simulink model "TSR_Scenario_005_cs"  (R2014b)
settings: Solver=ode5  SolverMode=SingleTasking  StartTime=0.0  StopTime=inf  FixedStep=1/100  RelTol=1e-3
PreLoadFcn:
  | mbxruntime.callbacks.PreLoadFcn(bdroot);
  | check_NUTS_defined;
  | 
  | assignin('base',['model_closed_' bdroot],false);
  | 
  | addpath('../includes_TSR/includes_TSR');
  | 
  | switch version('-release')
  | case {'2010a', '2010b', '2011a'}
  | addpath('../includes_TSR/ML2010b');
  | otherwise
  | addpath('../includes_TSR/ML2011b');
  | end
PostLoadFcn:
  | mbxruntime.callbacks.PostLoadFcn(bdroot);
InitFcn:
  | mbxruntime.callbacks.InitFcn(bdroot);
StartFcn:
  | mbxruntime.callbacks.StartFcn(bdroot);
StopFcn:
  | mbxruntime.callbacks.StopFcn(bdroot);
model workspace: external: MAT-File .\TSR_Scenario_005_cs_hws.mat (data not in the file)
undefined symbols (not defined in the file or in its folder): InitImageOutputDir, mbxruntime, OrientationPitch, OrientationRoll, PositionX, PositionY, PositionZ, tabledata, warningInitialVelocity, x0
undefined symbols (not defined in the file): SteeringColumn, SteeringWheel, TSR_Scenario_005_cs_00431f954bf6ed0a, TSR_Scenario_005_cs_02a6645fe307ce96, TSR_Scenario_005_cs_0e0d17e780cba748, TSR_Scenario_005_cs_0f94700004e304be, TSR_Scenario_005_cs_13e63084604f23c5, TSR_Scenario_005_cs_18da76569b226b1d, TSR_Scenario_005_cs_19a09eb0dceaf389, TSR_Scenario_005_cs_1d6b1ecf339da803, TSR_Scenario_005_cs_219485daa5a5d171, TSR_Scenario_005_cs_221c03cfb0670d1a, TSR_Scenario_005_cs_22611db63f83df91, TSR_Scenario_005_cs_24324341e1f0fdeb, TSR_Scenario_005_cs_248b5be6aaeb4a32, TSR_Scenario_005_cs_26d69342f02903e6, TSR_Scenario_005_cs_28d4639b4eb6a924, TSR_Scenario_005_cs_2a50646ef6121283, TSR_Scenario_005_cs_2addef8764f78195, TSR_Scenario_005_cs_2c78bb6e92f1c73d, TSR_Scenario_005_cs_330b013c7926b8c0, TSR_Scenario_005_cs_33ac55a3a4bfafc5, TSR_Scenario_005_cs_33d6442482a921b6, TSR_Scenario_005_cs_36fcc85960c1dc31, TSR_Scenario_005_cs_38acb22310967a91, TSR_Scenario_005_cs_3e8855054a9c05f5, TSR_Scenario_005_cs_43d01b44652f0f38, TSR_Scenario_005_cs_43d19ecb630bd754, TSR_Scenario_005_cs_4487c76a87b8c5f1, TSR_Scenario_005_cs_44ceee846c318dfb, TSR_Scenario_005_cs_450a3683cbfdd730, TSR_Scenario_005_cs_464618e49e37493a, TSR_Scenario_005_cs_4880b38df4698ab1, TSR_Scenario_005_cs_4a2b3c7d0abca22e, TSR_Scenario_005_cs_4bd204b8239d5406, TSR_Scenario_005_cs_4de8d67ffbf74a19, TSR_Scenario_005_cs_4f6170ee339e194e, TSR_Scenario_005_cs_50430c8166448bfc, TSR_Scenario_005_cs_53c8f6734eaacbd2, TSR_Scenario_005_cs_543db9a2ff458ebe, TSR_Scenario_005_cs_57976f30ab2edad5, TSR_Scenario_005_cs_5922fccf31372278, TSR_Scenario_005_cs_5a258c940bbe826b, TSR_Scenario_005_cs_6087cc283675db35, TSR_Scenario_005_cs_6246b869963d4acb, TSR_Scenario_005_cs_6352b9f9b72630f9, TSR_Scenario_005_cs_6559b64eceddc3ca, TSR_Scenario_005_cs_6832a8ea8fa66aa4, TSR_Scenario_005_cs_696d53dba69844e5, TSR_Scenario_005_cs_6cabbb37c4ac2dd1, TSR_Scenario_005_cs_6d528aa494c8a952, TSR_Scenario_005_cs_6d945b49f7234fd2, TSR_Scenario_005_cs_6e2ebc771acb2455, TSR_Scenario_005_cs_7897f864ad990cf0, TSR_Scenario_005_cs_7978c65fd141f076, TSR_Scenario_005_cs_7a9ba94120bbe2c7, TSR_Scenario_005_cs_7b108592703c2dc5, TSR_Scenario_005_cs_7cd2f5b09394b811, TSR_Scenario_005_cs_7e1904d085d8f37f, TSR_Scenario_005_cs_7e555208507e0618 ... (+95)
libraries: simulink_extras x59, PreScanSimulinkLibrary x43, simulink x29
(part 3 of 24)

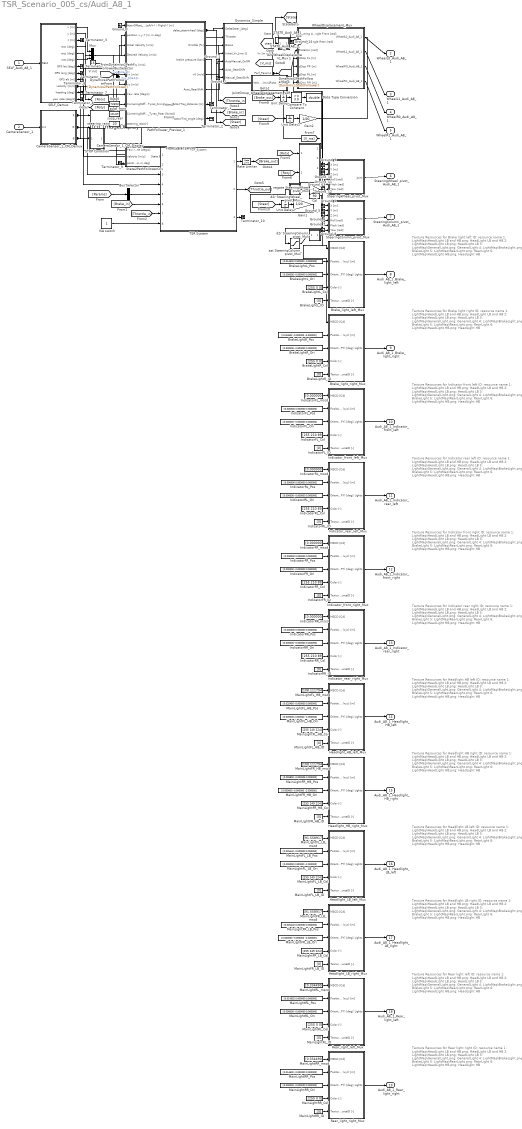
== system TSR_Scenario_005_cs/Audi_A8_1 ==
  note: Texture Resources for Brake light left
      |
      | ID: resource name
      | 1: LightMap\HeadLight LB and HB.png: HeadLight LB and HB
      | 2: LightMap\HeadLight LB.png: HeadLight LB
      | 3: LightMap\GeneralLight.png: GeneralLight
      | 4: LightMap\BrakeLight.png: BrakeLight
      | 5: LightMap\RearLight.png: RearLight
      | 6: LightMap\HeadLight HB.png: HeadLight HB
  note: Texture Resources for Brake light right
      |
      | ID: resource name
      | 1: LightMap\HeadLight LB and HB.png: HeadLight LB and HB
      | 2: LightMap\HeadLight LB.png: HeadLight LB
      | 3: LightMap\GeneralLight.png: GeneralLight
      | 4: LightMap\BrakeLight.png: BrakeLight
      | 5: LightMap\RearLight.png: RearLight
      | 6: LightMap\HeadLight HB.png: HeadLight HB
  note: Texture Resources for Indicator front left
      |
      | ID: resource name
      | 1: LightMap\HeadLight LB and HB.png: HeadLight LB and HB
      | 2: LightMap\HeadLight LB.png: HeadLight LB
      | 3: LightMap\GeneralLight.png: GeneralLight
      | 4: LightMap\BrakeLight.png: BrakeLight
      | 5: LightMap\RearLight.png: RearLight
      | 6: LightMap\HeadLight HB.png: HeadLight HB
  note: Texture Resources for Indicator rear left
      |
      | ID: resource name
      | 1: LightMap\HeadLight LB and HB.png: HeadLight LB and HB
      | 2: LightMap\HeadLight LB.png: HeadLight LB
      | 3: LightMap\GeneralLight.png: GeneralLight
      | 4: LightMap\BrakeLight.png: BrakeLight
      | 5: LightMap\RearLight.png: RearLight
      | 6: LightMap\HeadLight HB.png: HeadLight HB
  note: Texture Resources for Indicator front right
      |
      | ID: resource name
      | 1: LightMap\HeadLight LB and HB.png: HeadLight LB and HB
      | 2: LightMap\HeadLight LB.png: HeadLight LB
      | 3: LightMap\GeneralLight.png: GeneralLight
      | 4: LightMap\BrakeLight.png: BrakeLight
      | 5: LightMap\RearLight.png: RearLight
      | 6: LightMap\HeadLight HB.png: HeadLight HB
  note: Texture Resources for Indicator rear right
      |
      | ID: resource name
      | 1: LightMap\HeadLight LB and HB.png: HeadLight LB and HB
      | 2: LightMap\HeadLight LB.png: HeadLight LB
      | 3: LightMap\GeneralLight.png: GeneralLight
      | 4: LightMap\BrakeLight.png: BrakeLight
      | 5: LightMap\RearLight.png: RearLight
      | 6: LightMap\HeadLight HB.png: HeadLight HB
  note: Texture Resources for Headlight HB left
      |
      | ID: resource name
      | 1: LightMap\HeadLight LB and HB.png: HeadLight LB and HB
      | 2: LightMap\HeadLight LB.png: HeadLight LB
      | 3: LightMap\GeneralLight.png: GeneralLight
      | 4: LightMap\BrakeLight.png: BrakeLight
      | 5: LightMap\RearLight.png: RearLight
      | 6: LightMap\HeadLight HB.png: HeadLight HB
  note: Texture Resources for Headlight HB right
      |
      | ID: resource name
      | 1: LightMap\HeadLight LB and HB.png: HeadLight LB and HB
      | 2: LightMap\HeadLight LB.png: HeadLight LB
      | 3: LightMap\GeneralLight.png: GeneralLight
      | 4: LightMap\BrakeLight.png: BrakeLight
      | 5: LightMap\RearLight.png: RearLight
      | 6: LightMap\HeadLight HB.png: HeadLight HB
  note: Texture Resources for Headlight LB left
      |
      | ID: resource name
      | 1: LightMap\HeadLight LB and HB.png: HeadLight LB and HB
      | 2: LightMap\HeadLight LB.png: HeadLight LB
      | 3: LightMap\GeneralLight.png: GeneralLight
      | 4: LightMap\BrakeLight.png: BrakeLight
      | 5: LightMap\RearLight.png: RearLight
      | 6: LightMap\HeadLight HB.png: HeadLight HB
  note: Texture Resources for Headlight LB right
      |
      | ID: resource name
      | 1: LightMap\HeadLight LB and HB.png: HeadLight LB and HB
      | 2: LightMap\HeadLight LB.png: HeadLight LB
      | 3: LightMap\GeneralLight.png: GeneralLight
      | 4: LightMap\BrakeLight.png: BrakeLight
      | 5: LightMap\RearLight.png: RearLight
      | 6: LightMap\HeadLight HB.png: HeadLight HB
  note: Texture Resources for Rear light left
      |
      | ID: resource name
      | 1: LightMap\HeadLight LB and HB.png: HeadLight LB and HB
      | 2: LightMap\HeadLight LB.png: HeadLight LB
      | 3: LightMap\GeneralLight.png: GeneralLight
      | 4: LightMap\BrakeLight.png: BrakeLight
      | 5: LightMap\RearLight.png: RearLight
      | 6: LightMap\HeadLight HB.png: HeadLight HB
  note: Texture Resources for Rear light right
      |
      | ID: resource name
      | 1: LightMap\HeadLight LB and HB.png: HeadLight LB and HB
      | 2: LightMap\HeadLight LB.png: HeadLight LB
      | 3: LightMap\GeneralLight.png: GeneralLight
      | 4: LightMap\BrakeLight.png: BrakeLight
      | 5: LightMap\RearLight.png: RearLight
      | 6: LightMap\HeadLight HB.png: HeadLight HB
  SELF_Audi_A8_1 : Inport  Tag=inport/SelfPort  OutDataTypeStr=Bus: PRESCAN_SELFSENSORDATA  PortDimensions=1  SampleTime=1/100  BusOutputAsStruct=on
  CameraSensor_1 : Inport  Tag=inport/Camera/CameraSensor  Port=2  OutDataTypeStr=uint8  SampleTime=1/50  BusOutputAsStruct=on
  " " : Subsystem  mask{da=1.17, db=1.77, h=0.21, w=1.612}
      mask prompts: da "Distance to the front wheel from cars center of gravity [m]"; db "Distance to the back wheel from cars center of gravity [m]"; h "Center of gravity height [m]"; w "Width of the car [m]"
      mask init:
      | a  = sqrt( da*da + h*h );
      | b  = sqrt( db*db + h*h );
      | TW = sqrt( 0.25*w*w + h*h );
  BrakeLightL_Col : Constant  Tag=VisuLightConst  Value=[255 0 0]
  BrakeLightL_ID : Constant  Tag=VisuLightConst  Value=[0]
  BrakeLightL_Ori : Constant  Tag=VisuLightConst  Value=[0.000000 -0.000000 0.000000]
  BrakeLightL_Pos : Constant  Tag=VisuLightConst  Value=[0.014502 0.000000 -0.000000]
  BrakeLightR_Col : Constant  Tag=VisuLightConst  Value=[255 0 0]
  BrakeLightR_ID : Constant  Tag=VisuLightConst  Value=[0]
  BrakeLightR_Ori : Constant  Tag=VisuLightConst  Value=[0.000000 -0.000000 0.000000]
  BrakeLightR_Pos : Constant  Tag=VisuLightConst  Value=[0.014502 -0.000000 -0.000000]
  Brake_light_left_Mux : Subsystem  Tag=mux/ActiveLight  mask(PreScan User Interface: VisuActiveLight){}
      mask help:
      | The VisuActiveLight block provides a way for detailed animation of Light Sources, such as the indicator, brake, fog and main lights of a vehicle, or a light post.
      |
      | For more information, please click Help.
      settings: DeleteFcn=PreScanBlockDeleteFcn;
      mask Help: eval('openHelp(209)')
  Brake_light_right_Mux : Subsystem  Tag=mux/ActiveLight  mask(PreScan User Interface: VisuActiveLight){}
      mask help:
      | The VisuActiveLight block provides a way for detailed animation of Light Sources, such as the indicator, brake, fog and main lights of a vehicle, or a light post.
      |
      | For more information, please click Help.
      settings: DeleteFcn=PreScanBlockDeleteFcn;
      mask Help: eval('openHelp(209)')
  Bus Selector : BusSelector  OutputSignals=NEngine_[rpm]
  CameraSensor_1_CM_Demux : Subsystem  Tag=demux/Camera/Color  mask{SensorName=CameraSensor_1, hres=800, vres=600}
      mask prompts: SensorName "Sensor Name"; hres "Horizontal Resolution"; vres "Vertical Resolution"
      mask Help: eval('openHelp(457)')
      mask Display:
      | fprintf('MONO CAMERA:\n Color\n %s \n %d x %d px',SensorName,hres,vres)
      | port_label('output',1,'R')
      | port_label('output',2,'G')
      | port_label('output',3,'B')
  CameraSensor_1_CM_Display : M-S-Function  Tag=CameraSensor_Color_Display  InitFcn=InitImageOutputDir(gcb);  FunctionName=fcn_ImageDisplay  Parameters=SensorName EnableDisplay EnablePosition DisplayPosition FigureHandle SaveResults BitmapFormat TempOutputDir CameraType DataType  mask(PreScan Color Display Block){SensorName=CameraSensor_1, EnableDisplay=on, EnablePosition=off, DisplayPosition=[10 10 800 600], FigureHandle=21001, SaveResults=off, Format=PNG, TempOutputDir=0, CameraType=Mono, DataType=uint8}
      mask prompts: SensorName "User Specified: Title of Display"; EnableDisplay "Active"; EnablePosition "Set Display window position"; DisplayPosition "Display window position [xpos ypos width height]"; FigureHandle "Unique Handle"; SaveResults "Save results"; TempOutputDir "OutputDir"; CameraType "Camera Type"; DataType "Image Data Type"
      mask help: This block displays the RGB output of a PreScan camera sensor.
      mask init:
      | if EnableDisplay
      |     EnableString='';
      |     EnableColor='gray';
      | else
      |     EnableString='INACTIVE';
      |     EnableColor='red';
      | end
      | switch Format
      |     case 1
      |         BitmapFormat = 'png';
      |     case 2
      |         BitmapFormat = 'bmp';
      |     case 3
      |         BitmapFormat = 'jpg';
      | end 
      | if CameraType==1
      |     CameraTypeName='MONO';
      |     PortNumber=0;
      | else
      |     CameraTypeName='STEREO';
      |     PortNumber=3;
      | end
      settings: CopyFcn=CopyFcnDisplay  DeleteFcn=PreScanBlockDeleteFcn;  ModelCloseFcn=fcn_ImageDisplay_ModelCloseFcn
      mask Help: eval('openHelp(457)')
      mask Callback EnablePosition:
      | MV=get_param(gcb,'MaskVisibilities');
      | if strcmp(get_param(gcb,'EnablePosition'),'on')
      |     MV{4}='on';
      | else
      |     MV{4}='off';
      | end
      | set_param(gcb,'MaskVisibilities',MV);
      | clear MV;
      mask TypeOptions Format: PNG | BMP | JPG
      mask TypeOptions CameraType: Mono | Stereo
      mask TypeOptions DataType: uint8 | single
      mask Display:
      | color(EnableColor);
      | fprintf('%s\n DISPLAY:\n Color \n %s',EnableString,SensorName)
      | port_label('input',1,'R')
      | port_label('input',2,'G')
      | port_label('input',3,'B')
      | port_label('input',PortNumber+1,'R')
      | port_label('input',PortNumber+2,'G')
      | port_label('input',PortNumber+3,'B')
  Col : Constant  Value=90
  Compare To Constant : simulink/Logic and Bit Operations/Compare To Constant  relop=>=  const=3.0  OutDataTypeStr=boolean
  Data Type Conversion : DataTypeConversion  OutDataTypeStr=double
  Dynamics_Simple : Subsystem  Tag=Simple_Vehicle_Dynamics  mask(PreScan Block: Simple Dynamics){TimeStep=1/100, ComputationMode=Continuous_Time, initialX=TSR_Scenario_005_cs_Audi_A8_1_Dynamics_Simple_initialX, initialY=TSR_Scenario_005_cs_Audi_A8_1_Dynamics_Simple_initialY, initialZ=TSR_Scenario_005_cs_Audi_A8_1_Dynamics_Simple_initialZ, initialRoll=TSR_Scenario_005_cs_Audi_A8_1_Dynamics_Simple_initialRoll, initialPitch=TSR_Scenario_005_cs_Audi_A8_1_Dynamics_Simple_initialPitch, initialYaw=TSR_Scenario_005_cs_Audi_A8_1_Dynamics_Simple_initialYaw}
      mask prompts: TimeStep "Auto assigned: Time Step [s]"; ComputationMode "Computation mode:"; initialX "Ini x-position VEHICLE wrt GLOBAL axis system [m]"; initialY "Ini y-position VEHICLE wrt GLOBAL axis system [m]"; initialZ "Ini z-position VEHICLE wrt GLOBAL axis system [m]"; initialRoll "Ini roll-angle BODY wrt VEHICLE axis system [deg]"; initialPitch "Ini pitch-angle BODY wrt VEHICLE axis system [deg]"; initialYaw "Ini yaw-angle VEHICLE wrt GLOBAL axis system [deg]"
      mask help:
      | The Simple Dynamics Model is selected in the GUI to simulate vehicle dynamics behavior.
      |
      | The Simple Dynamics Model is completely open to the user. The parameters of this model can be set in the Simple Dynamics dialog in the GUI.
      |
      | For more information, please click Help.
      mask init:
      | p = SimpleDyn_pars;
      settings: DeleteFcn=PreScanBlockDeleteFcn;
      mask Help: eval('openHelp(220)')
      mask Display:
      | image(imread('SimpleDyn.png'))
      | port_label('input', 1, '{\delta}_S_t_ _e_e_r [deg]','texmode','on')
      | port_label('input', 2, 'Throttle [%]')
      | port_label('input', 3, 'Brake Pres [bar]')
      | port_label('input', 4, 'V_0 [ms-1]','texmode','on')
      | port_label('input', 5, 'Auto=[0]/Manual=[1]')
      | port_label('input', 6, 'Auto_GearShift')
      | port_label('input', 7, 'Manual_GearShift')
      | port_label('output', 1, 'State')
      | port_label('output', 2, 'Vx [ms-1]')
      | port_label('output', 3, 'Perf Params')
  FromDynamics2PathFollowerBusSelector : BusSelector  OutputSignals=vx_[ms-1],vy_[ms-1]
  Gain1 : Gain  Gain=1/20
  Gain2 : Gain  Gain=1/20
  Ground_{1..14} (14 alike) : Ground
  Headlight_HB_left_Mux : Subsystem  Tag=mux/ActiveLight  mask(PreScan User Interface: VisuActiveLight){}
      mask help:
      | The VisuActiveLight block provides a way for detailed animation of Light Sources, such as the indicator, brake, fog and main lights of a vehicle, or a light post.
      |
      | For more information, please click Help.
      settings: DeleteFcn=PreScanBlockDeleteFcn;
      mask Help: eval('openHelp(209)')
  Headlight_HB_right_Mux : Subsystem  Tag=mux/ActiveLight  mask(PreScan User Interface: VisuActiveLight){}
      mask help:
      | The VisuActiveLight block provides a way for detailed animation of Light Sources, such as the indicator, brake, fog and main lights of a vehicle, or a light post.
      |
      | For more information, please click Help.
      settings: DeleteFcn=PreScanBlockDeleteFcn;
      mask Help: eval('openHelp(209)')
  Headlight_LB_left_Mux : Subsystem  Tag=mux/ActiveLight  mask(PreScan User Interface: VisuActiveLight){}
      mask help:
      | The VisuActiveLight block provides a way for detailed animation of Light Sources, such as the indicator, brake, fog and main lights of a vehicle, or a light post.
      |
      | For more information, please click Help.
      settings: DeleteFcn=PreScanBlockDeleteFcn;
      mask Help: eval('openHelp(209)')
  Headlight_LB_right_Mux : Subsystem  Tag=mux/ActiveLight  mask(PreScan User Interface: VisuActiveLight){}
      mask help:
      | The VisuActiveLight block provides a way for detailed animation of Light Sources, such as the indicator, brake, fog and main lights of a vehicle, or a light post.
      |
      | For more information, please click Help.
      settings: DeleteFcn=PreScanBlockDeleteFcn;
      mask Help: eval('openHelp(209)')
  ISA switch : Constant
  IndicatorFL_Col : Constant  Tag=VisuLightConst  Value=[255 210 89]
  IndicatorFL_ID : Constant  Tag=VisuLightConst  Value=[0]
  IndicatorFL_Ori : Constant  Tag=VisuLightConst  Value=[0.000000 -0.000000 0.000000]
  IndicatorFL_Pos : Constant  Tag=VisuLightConst  Value=[0.000000 0.000000 0.000000]
  IndicatorFL_mscd : Constant  Tag=VisuLightConst  Value=[0.000000]
  IndicatorFR_Col : Constant  Tag=VisuLightConst  Value=[255 210 89]
  IndicatorFR_ID : Constant  Tag=VisuLightConst  Value=[0]
  IndicatorFR_Ori : Constant  Tag=VisuLightConst  Value=[0.000000 -0.000000 0.000000]
  IndicatorFR_Pos : Constant  Tag=VisuLightConst  Value=[0.000000 0.000000 0.000000]
  IndicatorFR_mscd : Constant  Tag=VisuLightConst  Value=[0.000000]
  IndicatorRL_Col : Constant  Tag=VisuLightConst  Value=[255 210 89]
  IndicatorRL_ID : Constant  Tag=VisuLightConst  Value=[0]
  IndicatorRL_Ori : Constant  Tag=VisuLightConst  Value=[0.000000 -0.000000 0.000000]
  IndicatorRL_Pos : Constant  Tag=VisuLightConst  Value=[0.000000 0.000000 0.000000]
  IndicatorRL_mscd : Constant  Tag=VisuLightConst  Value=[0.000000]
  IndicatorRR_Col : Constant  Tag=VisuLightConst  Value=[255 210 89]
  IndicatorRR_ID : Constant  Tag=VisuLightConst  Value=[0]
  IndicatorRR_Ori : Constant  Tag=VisuLightConst  Value=[0.000000 -0.000000 0.000000]
  IndicatorRR_Pos : Constant  Tag=VisuLightConst  Value=[0.000000 0.000000 0.000000]
  IndicatorRR_mscd : Constant  Tag=VisuLightConst  Value=[0.000000]
  Indicator_front_left_Mux : Subsystem  Tag=mux/ActiveLight  mask(PreScan User Interface: VisuActiveLight){}
      mask help:
      | The VisuActiveLight block provides a way for detailed animation of Light Sources, such as the indicator, brake, fog and main lights of a vehicle, or a light post.
      |
      | For more information, please click Help.
      settings: DeleteFcn=PreScanBlockDeleteFcn;
      mask Help: eval('openHelp(209)')
  Indicator_front_right_Mux : Subsystem  Tag=mux/ActiveLight  mask(PreScan User Interface: VisuActiveLight){}
      mask help:
      | The VisuActiveLight block provides a way for detailed animation of Light Sources, such as the indicator, brake, fog and main lights of a vehicle, or a light post.
      |
      | For more information, please click Help.
      settings: DeleteFcn=PreScanBlockDeleteFcn;
      mask Help: eval('openHelp(209)')
  Indicator_rear_left_Mux : Subsystem  Tag=mux/ActiveLight  mask(PreScan User Interface: VisuActiveLight){}
      mask help:
      | The VisuActiveLight block provides a way for detailed animation of Light Sources, such as the indicator, brake, fog and main lights of a vehicle, or a light post.
      |
      | For more information, please click Help.
      settings: DeleteFcn=PreScanBlockDeleteFcn;
      mask Help: eval('openHelp(209)')
  Indicator_rear_right_Mux : Subsystem  Tag=mux/ActiveLight  mask(PreScan User Interface: VisuActiveLight){}
      mask help:
      | The VisuActiveLight block provides a way for detailed animation of Light Sources, such as the indicator, brake, fog and main lights of a vehicle, or a light post.
      |
      | For more information, please click Help.
      settings: DeleteFcn=PreScanBlockDeleteFcn;
      mask Help: eval('openHelp(209)')
  JointGroup_WheelDisplacement_V2R : Subsystem  Tag=mux/Wheels  mask(PreScan Velocity to Wheel Angle Block:){TimeStep=1/100, TireRadius=0.34}
      mask prompts: TimeStep "Auto Assigned: Time Step [s]"; TireRadius "Tire Radius [m]"
      settings: DeleteFcn=PreScanBlockDeleteFcn;
      mask Display: disp('Velocity\nto\nWheelAngle')
  MainLightFL_HB_Col : Constant  Tag=VisuLightConst  Value=[255 249 224]
  MainLightFL_HB_ID : Constant  Tag=VisuLightConst  Value=[0]
  MainLightFL_HB_Ori : Constant  Tag=VisuLightConst  Value=[0.000000 2.000000 -2.000000]
  MainLightFL_HB_Pos : Constant  Tag=VisuLightConst  Value=[0.025450 -0.000000 0.000000]
  MainLightFL_HB_mscd : Constant  Tag=VisuLightConst  Value=[108.111794]
  MainLightFL_LB_Col : Constant  Tag=VisuLightConst  Value=[255 249 224]
  MainLightFL_LB_ID : Constant  Tag=VisuLightConst  Value=[0]
  MainLightFL_LB_Ori : Constant  Tag=VisuLightConst  Value=[0.000000 2.000000 -2.000000]
  MainLightFL_LB_Pos : Constant  Tag=VisuLightConst  Value=[0.025440 -0.000000 0.000000]
  MainLightFL_LB_mscd : Constant  Tag=VisuLightConst  Value=[91.558917]
  MainLightFR_HB_Col : Constant  Tag=VisuLightConst  Value=[255 249 224]
  MainLightFR_HB_ID : Constant  Tag=VisuLightConst  Value=[0]
  MainLightFR_HB_Ori : Constant  Tag=VisuLightConst  Value=[0.000000 -0.000000 -2.000000]
  MainLightFR_HB_Pos : Constant  Tag=VisuLightConst  Value=[0.025800 -0.000006 0.000000]
  MainLightFR_HB_mscd : Constant  Tag=VisuLightConst  Value=[108.111794]
  MainLightFR_LB_Col : Constant  Tag=VisuLightConst  Value=[255 249 224]
  MainLightFR_LB_ID : Constant  Tag=VisuLightConst  Value=[0]
  MainLightFR_LB_Ori : Constant  Tag=VisuLightConst  Value=[0.000000 -0.000000 -2.000000]
  MainLightFR_LB_Pos : Constant  Tag=VisuLightConst  Value=[0.025440 0.000030 0.000000]
  MainLightFR_LB_mscd : Constant  Tag=VisuLightConst  Value=[91.558917]
  MainLightRL_Col : Constant  Tag=VisuLightConst  Value=[255 0 0]
  MainLightRL_ID : Constant  Tag=VisuLightConst  Value=[0]
  MainLightRL_Ori : Constant  Tag=VisuLightConst  Value=[0.000000 -0.000000 0.000000]
  MainLightRL_Pos : Constant  Tag=VisuLightConst  Value=[0.014502 0.000000 0.000000]
  MainLightRL_mscd : Constant  Tag=VisuLightConst  Value=[0.334490]
  MainLightRR_Col : Constant  Tag=VisuLightConst  Value=[255 0 0]
  MainLightRR_ID : Constant  Tag=VisuLightConst  Value=[0]
  MainLightRR_Ori : Constant  Tag=VisuLightConst  Value=[0.000000 -0.000000 0.000000]
  MainLightRR_Pos : Constant  Tag=VisuLightConst  Value=[0.014502 -0.000000 0.000000]
  MainLightRR_mscd : Constant  Tag=VisuLightConst  Value=[0.334490]
  Mux : Mux  Inputs=3
  PathFollower_Preview_1 : Subsystem  Tag=PathFollower_Preview  mask(PreScan Block: Path Follower with Preview){LongCtrl_P=20, LongCtrl_I=0.3, LongCtrl_D=3.065, LongCtrl_AWU=1, LongCtrlDefault_P=20, LongCtrlDefault_I=0.3, LongCtrlDefault_D=3.065, LongCtrlDefault_AWU=1, PathUniqueID=TSR_Scenario_005_cs_18da76569b226b1d, mass=1820, Jzz=3746, length_a=1.17, length_l=2.94, Angle_Max_SteeringWheel=500, PreviewTime=1, DelayTime=0.1, LowSpeedLimit=20, MaxSteeringRate=1200, CSSampleTime=1/100, PFIntegrationFrequency=100}
      mask prompts: LongCtrl_P "Longitudinal Controller P"; LongCtrl_I "Longitudinal Controller I"; LongCtrl_D "Longitudinal Controller D"; LongCtrl_AWU "Longitudinal Controller AWU"; PathUniqueID "Path Unique ID"; mass "Mass vehicle total [kg]"; Jzz "Inertia vehicle around yaw axis [kg m2]"; length_a "Distance between COG and front axle [m]"; length_l "Length of wheelbase [m]"; Angle_Max_SteeringWheel "Maximum steering wheel angle [deg]"; PreviewTime "Preview time [s]"; DelayTime "Delay time [s]"; LowSpeedLimit "Low-speed limit [km/h]"; MaxSteeringRate "Maximum steering wheel angle rate [deg/s]"; CSSampleTime "Compilation Sheet sample time [s]"; PFIntegrationFrequency "Lateral controller frequency [Hz]"
      mask help:
      | The Path Follower Model is selected in the GUI to simulate driver behavior.
      |
      | For more information, please click Help.
      mask init:
      | RefreshCounter = max(floor((1/CSSampleTime) / (PFIntegrationFrequency)), 1);
      | PathFollowerBlockPath = gcb;
      mask Help: eval('openHelp(233)')
      mask DialogControl Control2 Prompt: Reset PID parameters
      mask DialogControl Control2 Callback:
      | LongCtrlDefault_P = get_param(gcb,'LongCtrlDefault_P');
      | set_param(gcb,'LongCtrl_P',LongCtrlDefault_P);
      | 
      | LongCtrlDefault_I = get_param(gcb,'LongCtrlDefault_I');
      | set_param(gcb,'LongCtrl_I',LongCtrlDefault_I);
      | 
      | LongCtrlDefault_D = get_param(gcb,'LongCtrlDefault_D');
      | set_param(gcb,'LongCtrl_D',LongCtrlDefault_D);
      | 
      | LongCtrlDefault_AWU = get_param(gcb,'LongCtrlDefault_AWU');
      | set_param(gcb,'LongCtrl_AWU',LongCtrlDefault_AWU);
  Rate Limiter : RateLimiter  RisingSlewLimit=150  FallingSlewLimit=-150  SampleTimeMode=inherited
  Rear_light_left_Mux : Subsystem  Tag=mux/ActiveLight  mask(PreScan User Interface: VisuActiveLight){}
      mask help:
      | The VisuActiveLight block provides a way for detailed animation of Light Sources, such as the indicator, brake, fog and main lights of a vehicle, or a light post.
      |
      | For more information, please click Help.
      settings: DeleteFcn=PreScanBlockDeleteFcn;
      mask Help: eval('openHelp(209)')
  Rear_light_right_Mux : Subsystem  Tag=mux/ActiveLight  mask(PreScan User Interface: VisuActiveLight){}
      mask help:
      | The VisuActiveLight block provides a way for detailed animation of Light Sources, such as the indicator, brake, fog and main lights of a vehicle, or a light post.
      |
      | For more information, please click Help.
      settings: DeleteFcn=PreScanBlockDeleteFcn;
      mask Help: eval('openHelp(209)')
  SELF_Demux : Subsystem  Tag=demux/SelfPort  mask(PreScan Demux Block:){}
      mask help:
      | The SELF port shows (state) information of the actor itself. The outputs are position in the experiment's axis system and the GPS coordinates, and the object's absolute velocity and compass heading.
      |
      | For more information, please click Help.
      settings: DeleteFcn=PreScanBlockDeleteFcn;
      mask Help: eval('openHelp(462)')
      mask Display:
      | port_label('output',1,'x [m]')
      | port_label('output',2,'y [m]')
      | port_label('output',3,'z [m]','texmode','on')
      | port_label('output',4,'Rotx [deg]','texmode','on')
      | port_label('output',5,'Roty [deg]','texmode','on')
      | port_label('output',6,'Rotz [deg]','texmode','on')
      | port_label('output',7,'GPS lat [deg]','texmode','on')
      | port_label('output',8,'GPS long [deg]','texmode','on')
      | port_label('output',9,'GPS alt [m]','texmode','on')
      | port_label('output',10,'Velocity [m/s]')
      | port_label('output',11,'Heading [deg]')
      | port_label('output',12,'Yaw rate [deg/s]')
  STATE_Audi_A8_1_rc : RateTransition  Tag=mux_rc/StatePort  OutPortSampleTimeOpt=Inherit
  STOP Condition : Subsystem
  State2PathFollowerCnv : Subsystem  Tag=State2PFConnection/cnv
  SteeringColumn_pivot_Mux : Subsystem  Tag=mux/Joint  mask(PreScan Mux Block){DisplayName=SteeringColumn}
      mask prompts: DisplayName "Display Name"
      mask help:
      | This block simulates a generic joint used for generic models. This joint can be enabled/disabled from the GUI.
      |
      | For more information, please click Help.
      settings: DeleteFcn=PreScanBlockDeleteFcn;
      mask Help: eval('openHelp(254)')
  SteeringWheel_pivot_Mux : Subsystem  Tag=mux/Joint  mask(PreScan Mux Block){DisplayName=SteeringWheel}
      mask prompts: DisplayName "Display Name"
      mask help:
      | This block simulates a generic joint used for generic models. This joint can be enabled/disabled from the GUI.
      |
      | For more information, please click Help.
      settings: DeleteFcn=PreScanBlockDeleteFcn;
      mask Help: eval('openHelp(254)')
  TSR System : ModelReference  ModelNameDialog=TSR_System  SimulationMode=Normal  ModelReferenceVersion=1.1003  CopyOfModelName=TSR_System  DefaultDataLogging=off
  Terminator_{1..10} (10 alike) : Terminator
  Unit Delay : UnitDelay  SampleTime=-1
  Unit Delay1 : UnitDelay  SampleTime=-1
  Unit Delay2 : UnitDelay  SampleTime=-1
  V init : Constant  Value=15
  WheelDisplacement_Mux : Subsystem  Tag=mux/JointGroup  mask(JointGroup){}
      mask help:
      | The JointGroup allows to control several Joints in one go, as defined for this particular model.
      | For more information, look in the PreScan manual in the section "Model Preparation Tool" -> "Joint Groups"
      |
      | For more information on the Joints simulink interface, press Help.
      mask Help: eval('openHelp(254)')
  d2r SteeringColumn_pivot_Mux : Subsystem  mask(DegreesToRadians){}
      mask help: SimulinkBlocks:simulink_extras:DegreesToRadians_MD
      mask Help: web([docroot '/simulink/ref_extras/degreestoradians.html'])
      mask Display: disp('D2R')
  d2r SteeringWheel_pivot_Mux : Subsystem  mask(DegreesToRadians){}
      mask help: SimulinkBlocks:simulink_extras:DegreesToRadians_MD
      mask Help: web([docroot '/simulink/ref_extras/degreestoradians.html'])
      mask Display: disp('D2R')
  d2r WheelDisplacement_Mux 1 : Subsystem  mask(DegreesToRadians){}
      mask help: SimulinkBlocks:simulink_extras:DegreesToRadians_MD
      mask Help: web([docroot '/simulink/ref_extras/degreestoradians.html'])
      mask Display: disp('D2R')
  negate SteeringWheel_pivot_Mux : Gain  Gain=-1
  sat SteeringColumn_pivot_Mux : Saturate  UpperLimit=30  LowerLimit=-5
  steering_ratio : Constant  Tag=steering_ratio  Value=20
  susp_front : Constant  Tag=susp_front  Value=72653
  susp_rear : Constant  Tag=susp_rear  Value=121449
  STATE_Audi_A8_1_bus : Outport  Tag=outport/StatePort  OutDataTypeStr=Bus: PRESCAN_STATEACTUATORDATA  PortDimensions=1  SampleTime=1/100
  WheelL0_Audi_A8_1 : Outport  Tag=outport/JointActuator  Port=2  OutDataTypeStr=Bus: PRESCAN_POSE_DATA  SampleTime=1/100
  WheelL1_Audi_A8_1 : Outport  Tag=outport/JointActuator  Port=3  OutDataTypeStr=Bus: PRESCAN_POSE_DATA  SampleTime=1/100
  WheelR0_Audi_A8_1 : Outport  Tag=outport/JointActuator  Port=4  OutDataTypeStr=Bus: PRESCAN_POSE_DATA  SampleTime=1/100
  WheelR1_Audi_A8_1 : Outport  Tag=outport/JointActuator  Port=5  OutDataTypeStr=Bus: PRESCAN_POSE_DATA  SampleTime=1/100
  SteeringWheel_pivot_Audi_A8_1 : Outport  Tag=outport/JointActuator  Port=6  OutDataTypeStr=Bus: PRESCAN_POSE_DATA  SampleTime=1/100
  SteeringColumn_pivot_Audi_A8_1 : Outport  Tag=outport/JointActuator  Port=7  OutDataTypeStr=Bus: PRESCAN_POSE_DATA  SampleTime=1/100
  Audi_A8_1_Brake_light_left : Outport  Tag=outport/BrakeLightL  Port=8  OutDataTypeStr=Bus: PRESCAN_VISULIGHTACTUATOR_DATA  SampleTime=1/100
  Audi_A8_1_Brake_light_right : Outport  Tag=outport/BrakeLightR  Port=9  OutDataTypeStr=Bus: PRESCAN_VISULIGHTACTUATOR_DATA  SampleTime=1/100
  Audi_A8_1_Indicator_front_left : Outport  Tag=outport/IndicatorFL  Port=10  OutDataTypeStr=Bus: PRESCAN_VISULIGHTACTUATOR_DATA  SampleTime=1/100
  Audi_A8_1_Indicator_rear_left : Outport  Tag=outport/IndicatorRL  Port=11  OutDataTypeStr=Bus: PRESCAN_VISULIGHTACTUATOR_DATA  SampleTime=1/100
  Audi_A8_1_Indicator_front_right : Outport  Tag=outport/IndicatorFR  Port=12  OutDataTypeStr=Bus: PRESCAN_VISULIGHTACTUATOR_DATA  SampleTime=1/100
  Audi_A8_1_Indicator_rear_right : Outport  Tag=outport/IndicatorRR  Port=13  OutDataTypeStr=Bus: PRESCAN_VISULIGHTACTUATOR_DATA  SampleTime=1/100
  Audi_A8_1_Headlight_HB_left : Outport  Tag=outport/MainLightFL_HB  Port=14  OutDataTypeStr=Bus: PRESCAN_VISULIGHTACTUATOR_DATA  SampleTime=1/100
  Audi_A8_1_Headlight_HB_right : Outport  Tag=outport/MainLightFR_HB  Port=15  OutDataTypeStr=Bus: PRESCAN_VISULIGHTACTUATOR_DATA  SampleTime=1/100
  Audi_A8_1_Headlight_LB_left : Outport  Tag=outport/MainLightFL_LB  Port=16  OutDataTypeStr=Bus: PRESCAN_VISULIGHTACTUATOR_DATA  SampleTime=1/100
  Audi_A8_1_Headlight_LB_right : Outport  Tag=outport/MainLightFR_LB  Port=17  OutDataTypeStr=Bus: PRESCAN_VISULIGHTACTUATOR_DATA  SampleTime=1/100
  Audi_A8_1_Rear_light_left : Outport  Tag=outport/MainLightRL  Port=18  OutDataTypeStr=Bus: PRESCAN_VISULIGHTACTUATOR_DATA  SampleTime=1/100
  Audi_A8_1_Rear_light_right : Outport  Tag=outport/MainLightRR  Port=19  OutDataTypeStr=Bus: PRESCAN_VISULIGHTACTUATOR_DATA  SampleTime=1/100
  tag scope: view=global
  wires:
  [Rotx] -> " "/1(rotX [deg])
  [Roty] -> " "/2(rotY [deg])
  " "/1(zDisp FL [m]) -> WheelDisplacement_Mux/4(zDisp FL [m])
  " "/2(zDisp FR [m]) -> WheelDisplacement_Mux/5(zDisp FR [m])
  " "/3(zDisp RL [m]) -> WheelDisplacement_Mux/6(zDisp RL [m])
  " "/4(zDisp RR [m]) -> WheelDisplacement_Mux/7(zDisp RR [m])
  Bus Selector/1 -> TSR System/5
  TSR System/1 -> Rate Limiter/1
  Rate Limiter/1 -> [Brake_out]
  TSR System/2 -> [Throttle_out]
  [Brake_in] -> TSR System/6
  [Throttle_in] -> TSR System/7
  ISA switch/1 -> TSR System/8
  [Params] -> Bus Selector/1
  SELF_Demux/10(velocity [m/s]) -> TSR System/1, STOP Condition/1(In1)
  CameraSensor_1_CM_Demux/1(R) -> TSR System/2, CameraSensor_1_CM_Display/1
  CameraSensor_1_CM_Demux/2(G) -> TSR System/3, CameraSensor_1_CM_Display/2
  CameraSensor_1_CM_Demux/3(B) -> TSR System/4, CameraSensor_1_CM_Display/3
  Col/1 -> sat SteeringColumn_pivot_Mux/1
  sat SteeringColumn_pivot_Mux/1 -> d2r SteeringColumn_pivot_Mux/1(Degrees in)
  d2r SteeringColumn_pivot_Mux/1(Radians out) -> SteeringColumn_pivot_Mux/5(Pitch [rad])
  Compare To Constant/1 -> Data Type Conversion/1
  Unit Delay/1 -> Compare To Constant/1
  [Brake_out] -> Unit Delay/1
  Data Type Conversion/1 -> Brake_light_left_Mux/1(MSCD [Cd]), Brake_light_right_Mux/1(MSCD [Cd])
  [Steer] -> Unit Delay2/1
  Unit Delay2/1 -> Gain1/1
  Gain1/1 -> d2r SteeringWheel_pivot_Mux/1(Degrees in)
  d2r SteeringWheel_pivot_Mux/1(Radians out) -> negate SteeringWheel_pivot_Mux/1
  negate SteeringWheel_pivot_Mux/1 -> SteeringWheel_pivot_Mux/4(Roll [rad])
  [Brake_out] -> Dynamics_Simple/3(Brake)
  [Throttle_out] -> Dynamics_Simple/2(Throttle)
  [V_ms] -> JointGroup_WheelDisplacement_V2R/1(Velocity [m/s])
  [Steer] -> Unit Delay1/1
  Unit Delay1/1 -> Gain2/1
  Gain2/1 -> d2r WheelDisplacement_Mux 1/1(Degrees in)
  d2r WheelDisplacement_Mux 1/1(Radians out) -> WheelDisplacement_Mux/1(Steering Angle Front [rad])
  Dynamics_Simple/1(State) -> [view], STATE_Audi_A8_1_rc/1, [State]
  Dynamics_Simple/3(Perf_Params) -> [Params], [Dynamics2PathFollower]
  PathFollower_Preview_1/3(brake pressure [bar]) -> [Brake_in]
  PathFollower_Preview_1/2(throttle [%]) -> [Throttle_in]
  SELF_Demux/4(rotx [deg]) -> [Rotx]
  SELF_Demux/5(roty [deg]) -> [Roty]
  Dynamics_Simple/2(Vx [m s-1]) -> [V_ms]
  PathFollower_Preview_1/1(delta_steerwheel [deg]) -> [Steer], Dynamics_Simple/1(DeltaSteer_[deg])
  Mux/1 -> PathFollower_Preview_1/2(position x,y,Y [m,m,deg])
  SELF_Demux/1(x [m]) -> Mux/1
  SELF_Demux/2(y [m]) -> Mux/2
  SELF_Demux/6(rotz [deg]) -> Mux/3
  STOP Condition/1(Out1) -> PathFollower_Preview_1/4(Desired Velocity [m/s])
  V init/1 -> PathFollower_Preview_1/3(Initial Velocity [m/s])
  STATE_Audi_A8_1_rc/1 -> STATE_Audi_A8_1_bus/1
  SELF_Audi_A8_1/1 -> SELF_Demux/1(SELF)
  CameraSensor_1/1 -> CameraSensor_1_CM_Demux/1(In1)
  WheelDisplacement_Mux/1(WheelL0_Audi_A8_1) -> WheelL0_Audi_A8_1/1
  WheelDisplacement_Mux/2(WheelL1_Audi_A8_1) -> WheelL1_Audi_A8_1/1
  WheelDisplacement_Mux/3(WheelR0_Audi_A8_1) -> WheelR0_Audi_A8_1/1
  WheelDisplacement_Mux/4(WheelR1_Audi_A8_1) -> WheelR1_Audi_A8_1/1
  JointGroup_WheelDisplacement_V2R/1(Rotation [rad]) -> WheelDisplacement_Mux/3(Rotation [rad])
  SteeringWheel_pivot_Mux/1(Joint) -> SteeringWheel_pivot_Audi_A8_1/1
  SteeringColumn_pivot_Mux/1(Joint) -> SteeringColumn_pivot_Audi_A8_1/1
  Brake_light_left_Mux/1(Lights) -> Audi_A8_1_Brake_light_left/1
  BrakeLightL_Pos/1 -> Brake_light_left_Mux/2(Position (xyz) [m])
  BrakeLightL_Ori/1 -> Brake_light_left_Mux/3(Orientation (RPY) [deg])
  BrakeLightL_Col/1 -> Brake_light_left_Mux/4(Color [-])
  BrakeLightL_ID/1 -> Brake_light_left_Mux/5(TextureResourceID [-])
  Brake_light_right_Mux/1(Lights) -> Audi_A8_1_Brake_light_right/1
  BrakeLightR_Pos/1 -> Brake_light_right_Mux/2(Position (xyz) [m])
  BrakeLightR_Ori/1 -> Brake_light_right_Mux/3(Orientation (RPY) [deg])
  BrakeLightR_Col/1 -> Brake_light_right_Mux/4(Color [-])
  BrakeLightR_ID/1 -> Brake_light_right_Mux/5(TextureResourceID [-])
  Indicator_front_left_Mux/1(Lights) -> Audi_A8_1_Indicator_front_left/1
  IndicatorFL_mscd/1 -> Indicator_front_left_Mux/1(MSCD [Cd])
  IndicatorFL_Pos/1 -> Indicator_front_left_Mux/2(Position (xyz) [m])
  IndicatorFL_Ori/1 -> Indicator_front_left_Mux/3(Orientation (RPY) [deg])
  IndicatorFL_Col/1 -> Indicator_front_left_Mux/4(Color [-])
  IndicatorFL_ID/1 -> Indicator_front_left_Mux/5(TextureResourceID [-])
  Indicator_rear_left_Mux/1(Lights) -> Audi_A8_1_Indicator_rear_left/1
  IndicatorRL_mscd/1 -> Indicator_rear_left_Mux/1(MSCD [Cd])
  IndicatorRL_Pos/1 -> Indicator_rear_left_Mux/2(Position (xyz) [m])
  IndicatorRL_Ori/1 -> Indicator_rear_left_Mux/3(Orientation (RPY) [deg])
  IndicatorRL_Col/1 -> Indicator_rear_left_Mux/4(Color [-])
  IndicatorRL_ID/1 -> Indicator_rear_left_Mux/5(TextureResourceID [-])
  Indicator_front_right_Mux/1(Lights) -> Audi_A8_1_Indicator_front_right/1
  IndicatorFR_mscd/1 -> Indicator_front_right_Mux/1(MSCD [Cd])
  IndicatorFR_Pos/1 -> Indicator_front_right_Mux/2(Position (xyz) [m])
  IndicatorFR_Ori/1 -> Indicator_front_right_Mux/3(Orientation (RPY) [deg])
  IndicatorFR_Col/1 -> Indicator_front_right_Mux/4(Color [-])
  IndicatorFR_ID/1 -> Indicator_front_right_Mux/5(TextureResourceID [-])
  Indicator_rear_right_Mux/1(Lights) -> Audi_A8_1_Indicator_rear_right/1
  IndicatorRR_mscd/1 -> Indicator_rear_right_Mux/1(MSCD [Cd])
  IndicatorRR_Pos/1 -> Indicator_rear_right_Mux/2(Position (xyz) [m])
  IndicatorRR_Ori/1 -> Indicator_rear_right_Mux/3(Orientation (RPY) [deg])
  IndicatorRR_Col/1 -> Indicator_rear_right_Mux/4(Color [-])
  IndicatorRR_ID/1 -> Indicator_rear_right_Mux/5(TextureResourceID [-])
  Headlight_HB_left_Mux/1(Lights) -> Audi_A8_1_Headlight_HB_left/1
  MainLightFL_HB_mscd/1 -> Headlight_HB_left_Mux/1(MSCD [Cd])
  MainLightFL_HB_Pos/1 -> Headlight_HB_left_Mux/2(Position (xyz) [m])
  MainLightFL_HB_Ori/1 -> Headlight_HB_left_Mux/3(Orientation (RPY) [deg])
  MainLightFL_HB_Col/1 -> Headlight_HB_left_Mux/4(Color [-])
  MainLightFL_HB_ID/1 -> Headlight_HB_left_Mux/5(TextureResourceID [-])
  Headlight_HB_right_Mux/1(Lights) -> Audi_A8_1_Headlight_HB_right/1
  MainLightFR_HB_mscd/1 -> Headlight_HB_right_Mux/1(MSCD [Cd])
  MainLightFR_HB_Pos/1 -> Headlight_HB_right_Mux/2(Position (xyz) [m])
  MainLightFR_HB_Ori/1 -> Headlight_HB_right_Mux/3(Orientation (RPY) [deg])
  MainLightFR_HB_Col/1 -> Headlight_HB_right_Mux/4(Color [-])
  MainLightFR_HB_ID/1 -> Headlight_HB_right_Mux/5(TextureResourceID [-])
  Headlight_LB_left_Mux/1(Lights) -> Audi_A8_1_Headlight_LB_left/1
  MainLightFL_LB_mscd/1 -> Headlight_LB_left_Mux/1(MSCD [Cd])
  MainLightFL_LB_Pos/1 -> Headlight_LB_left_Mux/2(Position (xyz) [m])
  MainLightFL_LB_Ori/1 -> Headlight_LB_left_Mux/3(Orientation (RPY) [deg])
  MainLightFL_LB_Col/1 -> Headlight_LB_left_Mux/4(Color [-])
  MainLightFL_LB_ID/1 -> Headlight_LB_left_Mux/5(TextureResourceID [-])
  Headlight_LB_right_Mux/1(Lights) -> Audi_A8_1_Headlight_LB_right/1
  MainLightFR_LB_mscd/1 -> Headlight_LB_right_Mux/1(MSCD [Cd])
  MainLightFR_LB_Pos/1 -> Headlight_LB_right_Mux/2(Position (xyz) [m])
  MainLightFR_LB_Ori/1 -> Headlight_LB_right_Mux/3(Orientation (RPY) [deg])
  MainLightFR_LB_Col/1 -> Headlight_LB_right_Mux/4(Color [-])
  MainLightFR_LB_ID/1 -> Headlight_LB_right_Mux/5(TextureResourceID [-])
  Rear_light_left_Mux/1(Lights) -> Audi_A8_1_Rear_light_left/1
  MainLightRL_mscd/1 -> Rear_light_left_Mux/1(MSCD [Cd])
  MainLightRL_Pos/1 -> Rear_light_left_Mux/2(Position (xyz) [m])
  MainLightRL_Ori/1 -> Rear_light_left_Mux/3(Orientation (RPY) [deg])
  MainLightRL_Col/1 -> Rear_light_left_Mux/4(Color [-])
  MainLightRL_ID/1 -> Rear_light_left_Mux/5(TextureResourceID [-])
  Rear_light_right_Mux/1(Lights) -> Audi_A8_1_Rear_light_right/1
  MainLightRR_mscd/1 -> Rear_light_right_Mux/1(MSCD [Cd])
  MainLightRR_Pos/1 -> Rear_light_right_Mux/2(Position (xyz) [m])
  MainLightRR_Ori/1 -> Rear_light_right_Mux/3(Orientation (RPY) [deg])
  MainLightRR_Col/1 -> Rear_light_right_Mux/4(Color [-])
  MainLightRR_ID/1 -> Rear_light_right_Mux/5(TextureResourceID [-])
  susp_front/1 -> PathFollower_Preview_1/9(CorneringStiffness_Tyres_Front [N/rad])
  susp_rear/1 -> PathFollower_Preview_1/10(CorneringStiffness_Tyres_Rear [N/rad])
  steering_ratio/1 -> PathFollower_Preview_1/11(steering_ratio[-])
  [State] -> State2PathFollowerCnv/1(State BUS)
  State2PathFollowerCnv/1(Yaw rate [deg/s]) -> PathFollower_Preview_1/8(Yaw rate [deg/s])
  State2PathFollowerCnv/2(velocity [m/s]) -> PathFollower_Preview_1/5(velocity [m/s])
  PathFollower_Preview_1/4(v0 [m/s]) -> Dynamics_Simple/4(Initial_Vx_[ms-1])
  PathFollower_Preview_1/5(Auto_GearShift) -> Dynamics_Simple/6(Auto_GearShift)
  FromDynamics2PathFollowerBusSelector/1 -> PathFollower_Preview_1/6(vx [m/s])  "<vx_[ms-1]>"
  FromDynamics2PathFollowerBusSelector/2 -> PathFollower_Preview_1/7(vy [m/s])  "<vy_[ms-1]>"
  [Dynamics2PathFollower] -> FromDynamics2PathFollowerBusSelector/1
  Ground_1/1 -> Dynamics_Simple/5(AutoManual_OnOff)
  Ground_2/1 -> Dynamics_Simple/7(Manual_GearShift)
  Ground_3/1 -> PathFollower_Preview_1/1(ActorOffset_Left(+) / Right(-) [m])
  PathFollower_Preview_1/6(Actor/Traj_distance [m]) -> Terminator_1/1
  PathFollower_Preview_1/7(Actor/Traj_angle [deg]) -> Terminator_2/1
  SELF_Demux/3(z [m]) -> Terminator_3/1
  SELF_Demux/7(GPS lat [deg]) -> Terminator_4/1
  SELF_Demux/8(GPS long [deg]) -> Terminator_5/1
  SELF_Demux/9(GPS alt [m]) -> Terminator_6/1
  SELF_Demux/11(heading [deg]) -> Terminator_7/1
  SELF_Demux/12(yaw rate [deg/s]) -> Terminator_8/1
  State2PathFollowerCnv/3(position x,y,Y [m,m,deg]) -> Terminator_9/1
  Ground_4/1 -> SteeringColumn_pivot_Mux/1(X [m])
  Ground_5/1 -> SteeringColumn_pivot_Mux/2(Y [m])
  Ground_6/1 -> SteeringColumn_pivot_Mux/3(Z [m])
  Ground_7/1 -> SteeringColumn_pivot_Mux/4(Roll [rad])
  Ground_8/1 -> SteeringColumn_pivot_Mux/6(Yaw [rad])
  Ground_9/1 -> SteeringWheel_pivot_Mux/1(X [m])
  Ground_10/1 -> SteeringWheel_pivot_Mux/2(Y [m])
  Ground_11/1 -> SteeringWheel_pivot_Mux/3(Z [m])
  Ground_12/1 -> SteeringWheel_pivot_Mux/5(Pitch [rad])
  Ground_13/1 -> SteeringWheel_pivot_Mux/6(Yaw [rad])
  TSR System/3 -> Terminator_10/1
  Ground_14/1 -> WheelDisplacement_Mux/2(Steering Angle Rear [rad])

== system TSR_Scenario_005_cs/Audi_A8_1_Brake_light_left ==
  Audi_A8_1_Brake_light_left : Inport  Tag=inport/BrakeLightL  OutDataTypeStr=Bus: PRESCAN_VISULIGHTACTUATOR_DATA  SampleTime=1/100  BusOutputAsStruct=on
  Actuator : S-Function  FunctionName=sfun_VisuLightActuator  Parameters=mbxruntime.parameters.convert(UniqueID), mbxruntime.parameters.convert(LightName), mbxruntime.parameters.convert(PivotName), mbxruntime.parameters.convert(TextureResources), mbxruntime.parameters.convert(ColorsObjectName), mbxruntime.parameters.convert(MeshOnColor), mbxruntime.parameters.convert(MeshOffColor),tabledata, TimeStep  EnableBusSupport=off  mask(PreScan Sink Block: VisuActiveLight){UniqueID=210, LightName=Audi_A8_1.LightActuator_0_BrakeLightRL_ActiveLight, PivotName=Audi_A8_1.BrakeLightL_pivot, TextureResources={ '1' 'LightMap\HeadLight LB and HB.png' '2' 'LightMap\HeadLight LB.png' '3' 'LightMap\GeneralLight.png' '4' 'LightMap\BrakeLight.png' '5' 'LightMap\RearLight.png' '6' 'LightMap\HeadLight HB.png'}, ColorsObjectName=Audi_A8_1.BrakeLightRL, MeshOnColor=[255    0    0  255  255    0    0  255  102  102  102  255  510    0    0  255], MeshOffColor=[255    0    0  255  255    0    0  255  102  102  102  255    0    0    0  255], TimeStep=1/100}
      mask prompts: UniqueID "Parent Unique Identifier"; LightName "Light"; PivotName "Pivot"; TextureResources "Texture Resources"; ColorsObjectName "Light Fixture Color Object"; MeshOnColor "Light Fixture On Color"; MeshOffColor "Light Fixture Off Color"; TimeStep "Simulink time step"
      mask help:
      | The VisuActiveLight block provides a way for detailed animation of Light Sources, such as the indicator, brake, fog and main lights of a vehicle, or a light post.
      |
      | For more information, please click Help.
      mask init:
      | [tabledata] = mbxruntime.parameters.table(UniqueID,LightName,PivotName,TextureResources,ColorsObjectName,MeshOnColor,MeshOffColor);
      mask Help: eval('openHelp(209)')
      mask Display: image(imread('HeadLight.png'))
  wires:
  Audi_A8_1_Brake_light_left/1 -> Actuator/1

== system TSR_Scenario_005_cs/Audi_A8_1_Brake_light_right ==
  Audi_A8_1_Brake_light_right : Inport  Tag=inport/BrakeLightR  OutDataTypeStr=Bus: PRESCAN_VISULIGHTACTUATOR_DATA  SampleTime=1/100  BusOutputAsStruct=on
  Actuator : S-Function  FunctionName=sfun_VisuLightActuator  Parameters=mbxruntime.parameters.convert(UniqueID), mbxruntime.parameters.convert(LightName), mbxruntime.parameters.convert(PivotName), mbxruntime.parameters.convert(TextureResources), mbxruntime.parameters.convert(ColorsObjectName), mbxruntime.parameters.convert(MeshOnColor), mbxruntime.parameters.convert(MeshOffColor),tabledata, TimeStep  EnableBusSupport=off  mask(PreScan Sink Block: VisuActiveLight){UniqueID=210, LightName=Audi_A8_1.LightActuator_1_BrakeLightRR_ActiveLight, PivotName=Audi_A8_1.BrakeLightR_pivot, TextureResources={ '1' 'LightMap\HeadLight LB and HB.png' '2' 'LightMap\HeadLight LB.png' '3' 'LightMap\GeneralLight.png' '4' 'LightMap\BrakeLight.png' '5' 'LightMap\RearLight.png' '6' 'LightMap\HeadLight HB.png'}, ColorsObjectName=Audi_A8_1.BrakeLightRR, MeshOnColor=[255    0    0  255  255    0    0  255  102  102  102  255  510    0    0  255], MeshOffColor=[255    0    0  255  255    0    0  255  102  102  102  255    0    0    0  255], TimeStep=1/100}
      mask prompts: UniqueID "Parent Unique Identifier"; LightName "Light"; PivotName "Pivot"; TextureResources "Texture Resources"; ColorsObjectName "Light Fixture Color Object"; MeshOnColor "Light Fixture On Color"; MeshOffColor "Light Fixture Off Color"; TimeStep "Simulink time step"
      mask help:
      | The VisuActiveLight block provides a way for detailed animation of Light Sources, such as the indicator, brake, fog and main lights of a vehicle, or a light post.
      |
      | For more information, please click Help.
      mask init:
      | [tabledata] = mbxruntime.parameters.table(UniqueID,LightName,PivotName,TextureResources,ColorsObjectName,MeshOnColor,MeshOffColor);
      mask Help: eval('openHelp(209)')
      mask Display: image(imread('HeadLight.png'))
  wires:
  Audi_A8_1_Brake_light_right/1 -> Actuator/1

== system TSR_Scenario_005_cs/Audi_A8_1_Headlight_HB_left ==
  Audi_A8_1_Headlight_HB_left : Inport  Tag=inport/MainLightFL_HB  OutDataTypeStr=Bus: PRESCAN_VISULIGHTACTUATOR_DATA  SampleTime=1/100  BusOutputAsStruct=on
  Actuator : S-Function  FunctionName=sfun_VisuLightActuator  Parameters=mbxruntime.parameters.convert(UniqueID), mbxruntime.parameters.convert(LightName), mbxruntime.parameters.convert(PivotName), mbxruntime.parameters.convert(TextureResources), mbxruntime.parameters.convert(ColorsObjectName), mbxruntime.parameters.convert(MeshOnColor), mbxruntime.parameters.convert(MeshOffColor),tabledata, TimeStep  EnableBusSupport=off  mask(PreScan Sink Block: VisuActiveLight){UniqueID=210, LightName=Audi_A8_1.LightActuator_10_MainLightFL_HB_ActiveLight, PivotName=Audi_A8_1.MainLightFL_HB_pivot, TextureResources={ '1' 'LightMap\HeadLight LB and HB.png' '2' 'LightMap\HeadLight LB.png' '3' 'LightMap\GeneralLight.png' '4' 'LightMap\BrakeLight.png' '5' 'LightMap\RearLight.png' '6' 'LightMap\HeadLight HB.png'}, ColorsObjectName=Audi_A8_1.MainLightFL_HB, MeshOnColor=[255  255  255    0  255  255  255    0  102  102  102  255  510  498  448  255], MeshOffColor=[255  255  255    0  255  255  255    0  102  102  102  255    0    0    0  255], TimeStep=1/100}
      mask prompts: UniqueID "Parent Unique Identifier"; LightName "Light"; PivotName "Pivot"; TextureResources "Texture Resources"; ColorsObjectName "Light Fixture Color Object"; MeshOnColor "Light Fixture On Color"; MeshOffColor "Light Fixture Off Color"; TimeStep "Simulink time step"
      mask help:
      | The VisuActiveLight block provides a way for detailed animation of Light Sources, such as the indicator, brake, fog and main lights of a vehicle, or a light post.
      |
      | For more information, please click Help.
      mask init:
      | [tabledata] = mbxruntime.parameters.table(UniqueID,LightName,PivotName,TextureResources,ColorsObjectName,MeshOnColor,MeshOffColor);
      mask Help: eval('openHelp(209)')
      mask Display: image(imread('HeadLight.png'))
  wires:
  Audi_A8_1_Headlight_HB_left/1 -> Actuator/1
